simulink model "read_write_test"  (R2023a)
settings: Solver=FixedStepAuto  StartTime=0.0  StopTime=30  RelTol=1e-3
settings Model: ExtModeTrigDuration=2  Creator=zapat  LastModifiedBy=zapat
settings OptimizationCC: EnhancedBackFolding=on  PassReuseOutputArgsAs=Individual arguments  ZeroExternalMemoryAtStartup=off  ZeroInternalMemoryAtStartup=off  MaxStackSize=64  OptimizeBlockOrder=speed  DifferentSizesBufferReuse=on  OptimizationCustomize=off  EfficientTunableParamExpr=on
settings DebuggingCC: ParameterTunabilityLossMsg=error
settings HardwareCC: ProdBitPerPointer=32  ProdBitPerSizeT=32  ProdBitPerPtrDiffT=32  ProdLargestAtomicInteger=Long  ProdLargestAtomicFloat=Double  ProdWordSize=32  ProdHWDeviceType=ARM Compatible->ARM Cortex  UseEmbeddedCoderFeatures=off  UseSimulinkCoderFeatures=off
settings SFSimCC: MATLABDynamicMemAlloc=off
settings RTWCC: Description=Embedded Coder  SystemTargetFile=ert.tlc  HardwareBoard=Arduino Nano 33 BLE Sense  TemplateMakefile=ert_default_tmf  Toolchain=Arduino ARM MBED
settings CodeAppCC: ForceParamTrailComments=on  IgnoreCustomStorageClasses=off  OperatorAnnotations=on  SimulinkDataObjDesc=on  SFDataObjDesc=on  InsertBlockDesc=on
settings ERTTargetCC: SupportContinuousTime=on  SupportNonInlinedSFcns=on  SupportVariableSizeSignals=on  ExtModeTransport=3  ExtModeStaticAlloc=on  ExtModeAutomaticAllocSize=off  ExtModeStaticAllocSize=65536  ExtModeMexFile=ext_xcp  ExtModeIntrfLevel=Level2 - Open

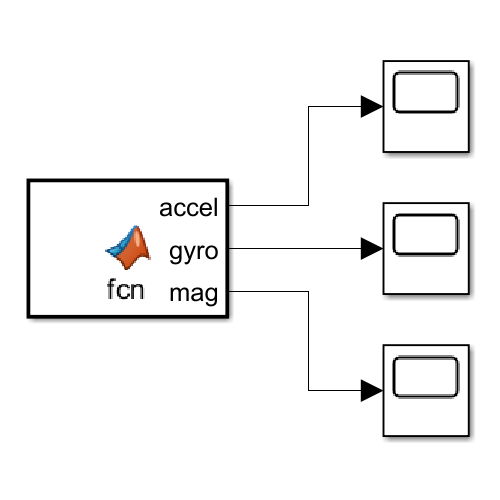
[thumbnail: Simulink's stored preview of the top-level diagram]
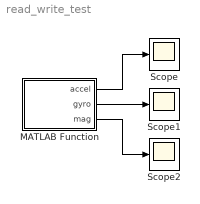
== system read_write_test ==
  MATLAB Function : MATLAB Function  TreatAsAtomicUnit=on
  Scope : Scope
  Scope1 : Scope
  Scope2 : Scope
  wires:
  MATLAB Function/2(gyro) -> Scope1/1
  MATLAB Function/1(accel) -> Scope/1
  MATLAB Function/3(mag) -> Scope2/1

== matlab function read_write_test/MATLAB Function ==
  data: accel output; gyro output; mag output
function [accel, gyro, mag] = fcn()
    persistent ble_device;    %automatically initialized to []
    persistent ble_imu;       %automatically initialized to []

    % Extrinsic declarations
    coder.extrinsic('ble');
    coder.extrinsic('characteristic');
    coder.extrinsic('read');

    % Connection information
    ARDUINO_NAME = 'Arduino Nanosat';
    IMU9DOF_UUID = "180C";
    IMU_UUID = "2A56"; % IMU (accel, gyro, mag)

    if isempty(ble_device)
        disp(['Connecting to BLE periferal ', ARDUINO_NAME, '...'])
        ble_device = ble(ARDUINO_NAME);
        disp('Accessing BLE characteristics...')
        ble_imu = characteristic(ble_device, IMU9DOF_UUID, IMU_UUID);
    end

    % Read IMU data
    accel = zeros(1, 3, 'single'); 
    gyro  = zeros(1, 3, 'single');
    mag   = zeros(1, 3, 'single');

    b = read(ble_imu); 
    imuData = typecast(uint8(b), 'single');

    accel(:) = imuData(1:3);
    gyro(:)  = imuData(4:6);
    mag(:)   = imuData(7:9);

end
